simulink model "MPC_observer"  (R2014b)
settings: Solver=ode45  StartTime=0.0  StopTime=T_sim  RelTol=1e-3
values from neighbouring files (symbols this model uses):
  C = [0, 1, 0, 0; 0, 0, 0, 1; -128.2, 128.2, 0, 0]    [cessna.m]
  N = 10    [cessna.m]
  Q_simulink = Q    [cessna.m]
  R = 10    [cessna.m]
  S_simulink = S    [cessna.m]
  set_point = [0; 0; 0; 0]    [cessna.m]
  sys_discrete = c2d(sys, Ts)    [cessna.m]
  sys_observer_discrete = c2d(sys_observer, Ts)    [cessna.m]
  Ts = 0.1    [cessna.m]
  u_max_simulink = u_max    (= 0.262)    [cessna.m]
  u_min_simulink = u_min    (= -0.262)    [cessna.m]
  uslopemax_simulink = u_slew_rate_max    (= 0.524)    [cessna.m]
  uslopemin_simulink = u_slew_rate_min    (= -0.524)    [cessna.m]
  x0 = [0; 0; 0; 10]    [cessna.m]
  x_max_simulink = [+inf, x2_max, +inf, x0(4) * (1 + overshot_fraction_h)]'    [cessna.m]
  x_min_simulink = [-inf, x2_min, -inf, - x0(4) * overshot_fraction_l]'    [cessna.m]
undefined symbols (not defined in the file or in its folder): MPC_controller
settings Model: Creator=lele  LastModifiedBy=lele

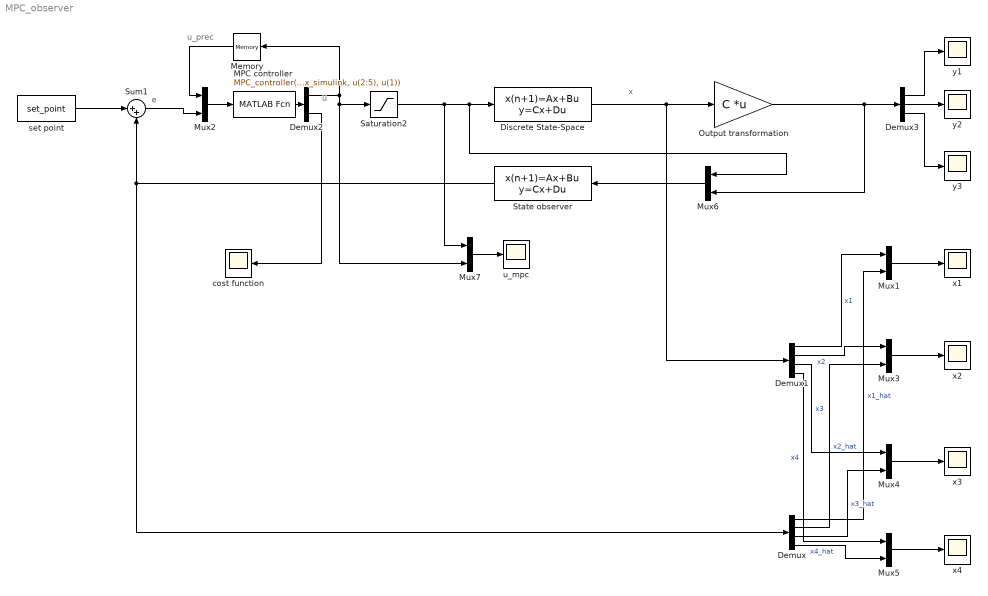
== system MPC_observer ==
  note: x
  note: u_prec
  note: u
  note: e
  Demux : Demux
  Demux1 : Demux
  Demux2 : Demux  Outputs=2
  Demux3 : Demux  Outputs=3
  Discrete State-Space : DiscreteStateSpace  A=sys_discrete.a  B=sys_discrete.b  C=eye(4)  D=zeros(4, 1)  X0=x0  SampleTime=Ts
  MPC controller : MATLABFcn  MATLABFcn=MPC_controller(sys_discrete, Q_simulink, R, S_simulink, N, u_min_simulink, u_max_simulink, uslopemin_simulink, uslopemax_simulink, x_min_simulink, x_max_simulink, u(2:5), u(1))  OutputDimensions=2  Output1D=off
  Memory : Memory
  Mux{1,3..7} (6 alike) : Mux  Inputs=2
  Mux2 : Mux  Inputs=[1 4]
  Output transformation : Gain  Gain=C  Multiplication=Matrix(K*u)
  Saturation2 : Saturate  UpperLimit=u_max_simulink  LowerLimit=u_min_simulink
  State observer : DiscreteStateSpace  A=sys_observer_discrete.a  B=sys_observer_discrete.b  C=sys_observer_discrete.c  D=sys_observer_discrete.d  X0=x0  SampleTime=Ts
  Sum1 : Sum  Inputs=|++
  cost function : Scope
      settings: ShowLegends=on  TimeRange=10  YMin=0  YMax=0.003  SaveName=ScopeData4
  set point : Constant  Value=set_point
  u_mpc : Scope
      settings: ShowLegends=on  SaveName=ScopeData2
  x{1..4} (4 alike) : Scope
      x1 settings: ShowLegends=on  TimeRange=10  SaveName=ScopeData6
      x2 settings: ShowLegends=on  SaveName=ScopeData7
      x3 settings: ShowLegends=on  SaveName=ScopeData8
      x4 settings: ShowLegends=on  YMin=-3  YMax=6  SaveName=ScopeData9
  y1 : Scope
      settings: ShowLegends=on  SaveName=ScopeData10
  y2 : Scope
      settings: ShowLegends=on  SaveName=ScopeData11
  y3 : Scope
      settings: ShowLegends=on  SaveName=ScopeData12
  wires:
  set point/1 -> Sum1/1
  Sum1/1 -> Mux2/2
  Mux2/1 -> MPC controller/1
  Memory/1 -> Mux2/1
  Saturation2/1 -> Mux7/1, Mux6/1, Discrete State-Space/1
  Mux7/1 -> u_mpc/1
  MPC controller/1 -> Demux2/1
  Demux2/1 -> Mux7/2, Saturation2/1, Memory/1
  Demux2/2 -> cost function/1
  Output transformation/1 -> Mux6/2, Demux3/1
  Demux3/1 -> y1/1
  Demux3/2 -> y2/1
  Demux3/3 -> y3/1
  Discrete State-Space/1 -> Demux1/1, Output transformation/1
  State observer/1 -> Sum1/2, Demux/1
  Demux1/1 -> Mux1/1  "x1"
  Demux/1 -> Mux1/2  "x1_hat"
  Demux1/2 -> Mux3/1  "x2"
  Demux/2 -> Mux3/2  "x2_hat"
  Demux1/3 -> Mux4/1  "x3"
  Demux/3 -> Mux4/2  "x3_hat"
  Demux1/4 -> Mux5/1  "x4"
  Demux/4 -> Mux5/2  "x4_hat"
  Mux1/1 -> x1/1
  Mux3/1 -> x2/1
  Mux4/1 -> x3/1
  Mux5/1 -> x4/1
  Mux6/1 -> State observer/1
